simulink model "relay"  (R2014b)
settings: Solver=ode3  StartTime=0.0  StopTime=0.1  FixedStep=0.001  RelTol=1e-3
values from neighbouring files (symbols this model uses):
  A = pi*dC^2/4    (= 3.84845100065e-05)    [relayModel.m]
  F_preload = 30e-3*g    (= 0.2943)    [relayModel.m]
  J = 8.5e-7    (= 8.5e-07)    [motorModel.m]    (also in relayModel.m = 3.89475e-08)
  k = 32e-3*g/1e-3    (= 313.92)    [relayModel.m]
  l = 12e-3    (= 0.012)    [relayModel.m]
  L1 = 70e-3    (= 0.07)    [relayModel.m]
  my0 = 4e-7*pi    (= 1.25663706144e-06)    [relayModel.m]
  myr = 100    [relayModel.m]
  nW = aW*bW/dW^2    (= 7200)    [relayModel.m]
  R = 288    [relayModel.m]
  x0 = 1e-3    (= 0.001)    [relayModel.m]
settings Model: Creator=Big Boy  LastModifiedBy=Big Boy

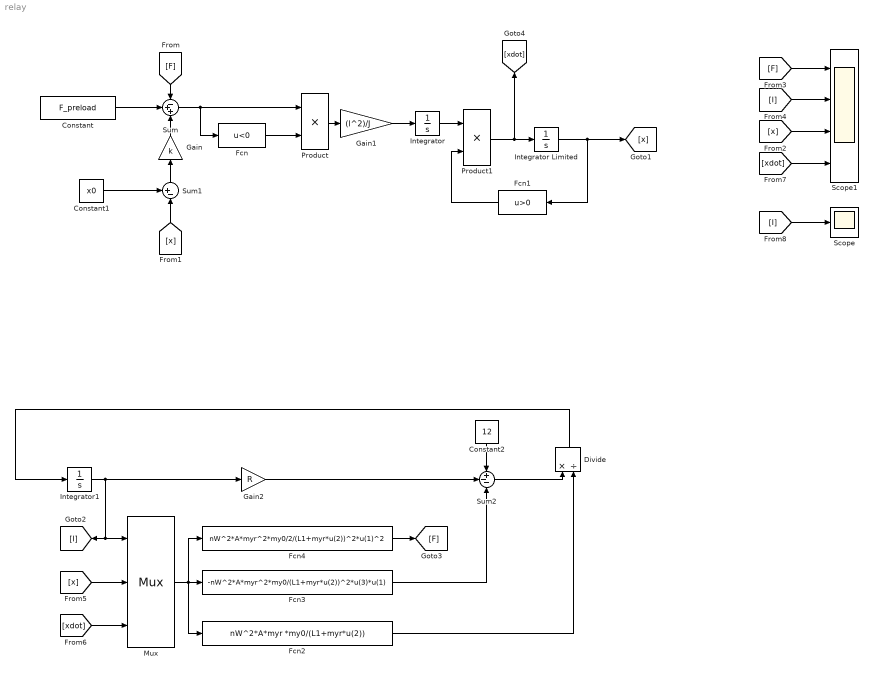
== system relay ==
  Constant : Constant  Value=F_preload
  Constant1 : Constant  Value=x0
  Constant2 : Constant  Value=12
  Divide : Product  Inputs=*/
  Fcn : Fcn  Expr=u<0
  Fcn1 : Fcn  Expr=u>0
  Fcn2 : Fcn  Expr=nW^2*A*myr *my0/(L1+myr*u(2))
  Fcn3 : Fcn  Expr=-nW^2*A*myr^2*my0/(L1+myr*u(2))^2*u(3)*u(1)
  Fcn4 : Fcn  Expr=nW^2*A*myr^2*my0/2/(L1+myr*u(2))^2*u(1)^2
  Gain : Gain  Gain=k
  Gain1 : Gain  Gain=(l^2)/J
  Gain2 : Gain  Gain=R
  Integrator : Integrator
  Integrator Limited : Integrator  InitialCondition=x0  LimitOutput=on  UpperSaturationLimit=1  LowerSaturationLimit=0
  Integrator1 : Integrator
  Mux : Mux  Inputs=3
  Product : Product
  Product1 : Product
  Scope : Scope
  Scope1 : Scope  NumInputPorts=4
      settings: YMin=-5~-5~-5~-5  YMax=5~5~5~5
  Sum : Sum  Inputs=-++
  Sum1 : Sum  Inputs=+-|
  Sum2 : Sum  Inputs=+--
  wires:
  Gain2/1 -> Sum2/2
  Constant2/1 -> Sum2/1
  Sum2/1 -> Divide/1
  Fcn3/1 -> Sum2/3
  Fcn4/1 -> [F]
  Fcn2/1 -> Divide/2
  Integrator1/1 -> [I], Mux/1, Gain2/1
  Divide/1 -> Integrator1/1
  [x] -> Mux/2
  [xdot] -> Mux/3
  Mux/1 -> Fcn2/1, Fcn4/1, Fcn3/1
  [F] -> Sum/1
  Constant/1 -> Sum/2
  Gain/1 -> Sum/3
  Sum/1 -> Product/1, Fcn/1
  Fcn/1 -> Product/2
  Product/1 -> Gain1/1
  Gain1/1 -> Integrator/1
  Product1/1 -> Integrator Limited/1, [xdot]
  Integrator/1 -> Product1/1
  Fcn1/1 -> Product1/2
  Integrator Limited/1 -> Fcn1/1, [x]
  [F] -> Scope1/1
  [I] -> Scope1/2
  [x] -> Scope1/3
  [xdot] -> Scope1/4
  [I] -> Scope/1
  [x] -> Sum1/2
  Constant1/1 -> Sum1/1
  Sum1/1 -> Gain/1
